simulink model "EMD_model_1"  (R2018b)
settings: Solver=ode45  StartTime=0.0  StopTime=setStopTime  FixedStep=0.0005  RelTol=1e-3  EnableMultiTasking=on
model workspace (MAT data in the model file):
  bodyAmp = 0
  bodyPhase = 0
  freq = 628.318530718
  headAmp = 0
  headPhase = 0
  imageData = [0.00228480667088 0.00685422825671 0.0114230745906 0.0159909622235 0.0205575077854 0.0251223280162 0.0296850397975 0.0342452601838 0.0388026064343 0.0433566960441 0.0479071467754 0.0524535766893 ... (8204 elements, 1x8204)]
  outputTimeList = [1 1.0001 1.0002 1.0003 1.0004 1.0005 1.0006 1.0007 1.0008 1.0009 1.001 1.0011 ... (101 elements, 1x101)]
  setStopTime = 1.01
  stimAmp = 15
  temporalFilt = 0.035
  timeConstant = 0.06
undefined symbols (not defined in the file): high_delay, low_delay, phot_a, photo_b
libraries: visionsources x1
(part 2 of 2)

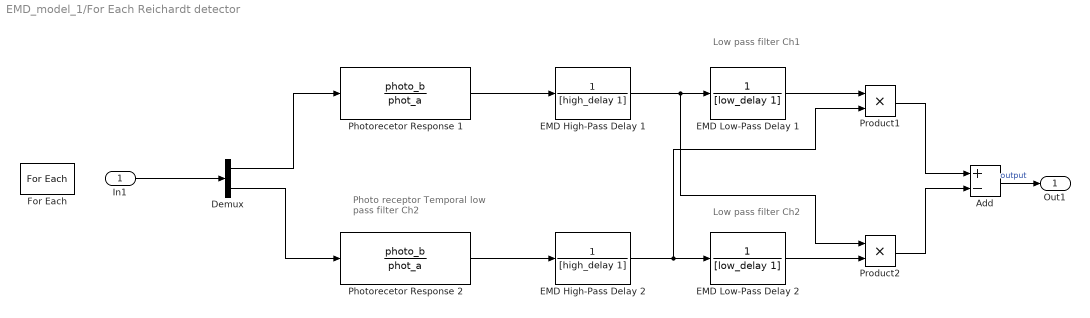
== system EMD_model_1/For Each Reichardt detector ==
  note: Photo receptor
      | Temporal low pass filter
      | Ch2
  note: Low pass filter
      | Ch1
  note: Low pass filter
      | Ch2
  In1 : Inport  Partition=on  PartitionDimension=1  PartitionWidth=1  PartitionOffset=0
  Add : Sum  Inputs=+-
  Demux : Demux  Outputs=2
  EMD High-Pass Delay 1 : TransferFcn  Denominator=[high_delay 1]
  EMD High-Pass Delay 2 : TransferFcn  Denominator=[high_delay 1]
  EMD Low-Pass Delay 1 : TransferFcn  Denominator=[low_delay 1]
  EMD Low-Pass Delay 2 : TransferFcn  Denominator=[low_delay 1]
  For Each : ForEach  DisableCoverage=on  IndexMode=One-based
  Photorecetor Response 1 : TransferFcn  Numerator=photo_b  Denominator=phot_a
  Photorecetor Response 2 : TransferFcn  Numerator=photo_b  Denominator=phot_a
  Product1 : Product  RndMeth=Zero
  Product2 : Product  RndMeth=Zero
  Out1 : Outport  ConcatenationDimension=1
  wires:
  EMD Low-Pass Delay 1/1 -> Product1/1
  Product1/1 -> Add/1
  Product2/1 -> Add/2
  EMD Low-Pass Delay 2/1 -> Product2/2
  Add/1 -> Out1/1  "output"
  In1/1 -> Demux/1
  Photorecetor Response 2/1 -> EMD High-Pass Delay 2/1
  Photorecetor Response 1/1 -> EMD High-Pass Delay 1/1
  Demux/1 -> Photorecetor Response 1/1
  Demux/2 -> Photorecetor Response 2/1
  EMD High-Pass Delay 1/1 -> EMD Low-Pass Delay 1/1, Product2/1
  EMD High-Pass Delay 2/1 -> EMD Low-Pass Delay 2/1, Product1/2

== matlab function EMD_model_1/sampleImage ==
  data: imageData input; intensity output double size=360,2; seenAngle input
function intensity = fcn(imageData,seenAngle)
%#codegen

imageWidth = length(imageData);

% Subsample with resolution of compound eye
sampleCoord = 0:359;
sampleCoord = sampleCoord + seenAngle;
sampleCoord = mod(sampleCoord,360);
temp        = interp1(linspace(0,360,imageWidth),imageData,sampleCoord);

% Create output signals
intensity = [temp(:), circshift(temp(:),-1)];
